simulink model "EffectofGain_TimeConstant_on_FirstOrderSys"  (R2024a)
settings: Solver=VariableStepAuto  StartTime=0.0  StopTime=10.0  RelTol=1e-3
settings Model: Creator=VICTUS  LastModifiedBy=VICTUS

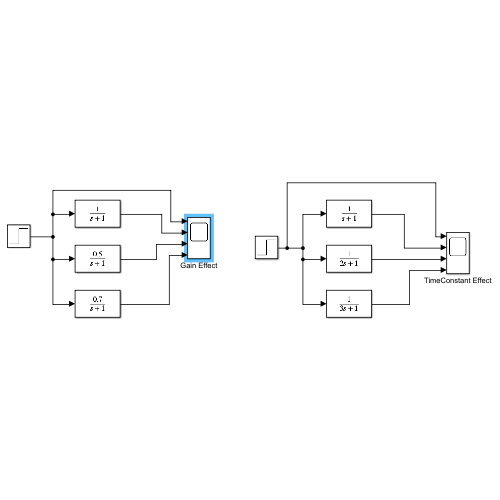
[thumbnail: Simulink's stored preview of the top-level diagram]
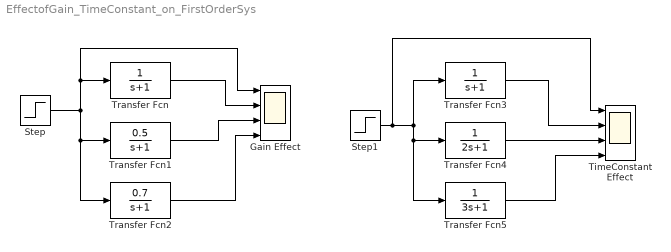
== system EffectofGain_TimeConstant_on_FirstOrderSys ==
  Gain Effect : Scope  NumInputPorts=4
  Step : Step  SampleTime=0
  Step1 : Step  SampleTime=0
  TimeConstant Effect : Scope  NumInputPorts=4
  Transfer Fcn : TransferFcn  Denominator=[1 1]
  Transfer Fcn1 : TransferFcn  Numerator=[0.5]  Denominator=[1 1]
  Transfer Fcn2 : TransferFcn  Numerator=[0.7]  Denominator=[1 1]
  Transfer Fcn3 : TransferFcn  Denominator=[1 1]
  Transfer Fcn4 : TransferFcn  Denominator=[2 1]
  Transfer Fcn5 : TransferFcn  Denominator=[3 1]
  wires:
  Step/1 -> Gain Effect/1, Transfer Fcn/1, Transfer Fcn2/1, Transfer Fcn1/1
  Transfer Fcn/1 -> Gain Effect/2
  Transfer Fcn1/1 -> Gain Effect/3
  Transfer Fcn2/1 -> Gain Effect/4
  Step1/1 -> TimeConstant Effect/1, Transfer Fcn3/1, Transfer Fcn5/1, Transfer Fcn4/1
  Transfer Fcn3/1 -> TimeConstant Effect/2
  Transfer Fcn4/1 -> TimeConstant Effect/3
  Transfer Fcn5/1 -> TimeConstant Effect/4
